simulink model "entryVehicle"  (R2024b)
settings: Solver=ode5  StartTime=startTime  StopTime=stopTime  FixedStep=stepTime  RelTol=1e-3
values from neighbouring files (symbols this model uses):
  acce_bias = [0; 0; 0]    [run_entryVehicle.m]
  acce_S = [0, 0, 0 ... (first row only)    [run_entryVehicle.m]
  alpha_0 = deg2rad(-23.82)    [run_entryVehicle.m]
  beta_0 = deg2rad(0.0)    [run_entryVehicle.m]
  chi_0 = deg2rad(90)    [run_entryVehicle.m]
  d_ref = 3.9    [run_entryVehicle.m]
  gamma_0 = deg2rad(-9.536)    [run_entryVehicle.m]
  H_s = 7050    [run_entryVehicle.m]
  I_xx = 5617.61    [run_entryVehicle.m]
  I_xz = 0    [run_entryVehicle.m]
  I_yy = 4454.62    [run_entryVehicle.m]
  I_zz = 4454.80    (= 4454.8)    [run_entryVehicle.m]
  lambda_0 = deg2rad(0)    [run_entryVehicle.m]
  m_0 = 4976    [run_entryVehicle.m]
  Mars_radius = 6371e3    (= 6371000)    [run_entryVehicle.m]
  p_0 = deg2rad(0)    [run_entryVehicle.m]
  Q0 = [Q1; Q2; Q3; Q4]    [get_Q0.m]    (also in run_entryVehicle.m = get_Q0(tau_0, lambda_0, chi_0, gamma_0, alpha_0, beta_0, sig)
  q_0 = deg2rad(0)    [run_entryVehicle.m]
  r0_eci = [x; y; z]    [getInitialECI.m]
  r_0 = deg2rad(0)    [run_entryVehicle.m]
  R_0 = 220e3 + Mars_radius    (= 6591000)    [run_entryVehicle.m]
  r_cm = [-0.137; 0; 1.8]    [run_entryVehicle.m]
  R_s = 287    [run_entryVehicle.m]
  rateGyro_bias = [0; 0; 0]    [run_entryVehicle.m]
  rateGyro_S = [0, 0, 0 ... (first row only)    [run_entryVehicle.m]
  rho_0 = 1.225    [run_entryVehicle.m]
  S_ref = 12    [run_entryVehicle.m]
  sigma_0 = deg2rad(100.)    [run_entryVehicle.m]
  specific_heat = 1.29    [run_entryVehicle.m]
  stepTime = 0.01    [run_entryVehicle.m]
  tau_0 = deg2rad(0)    [run_entryVehicle.m]
  v0_eci = T_ECI_NED * v_ned    [getInitialECI.m]
  V_0 = 11e3    (= 11000)    [run_entryVehicle.m]
undefined symbols (not defined in the file or in its folder): A_attitude, alpha_T_CD, alpha_T_CL, alpha_T_Cm, alpha_T_Cm_q, B_attitude, CD_T, CL_T, Cm_qT, Cm_T, K_lat, K_long, lateral_ref, longitudinal_ref, Mach_numbers_CD, Mach_numbers_CL, Mach_numbers_Cm, Mach_numbers_Cm_q, Mars_mu, my_max
libraries: simulink_extras x33, aerolibnav x2, simulink x1, SignalEditorBlockLib x1
(part 1 of 2)
settings Model: Creator=tester  LastModifiedBy=rafae

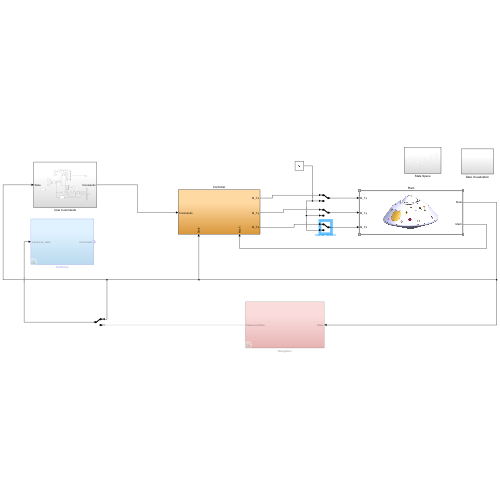
[thumbnail: Simulink's stored preview of the top-level diagram]
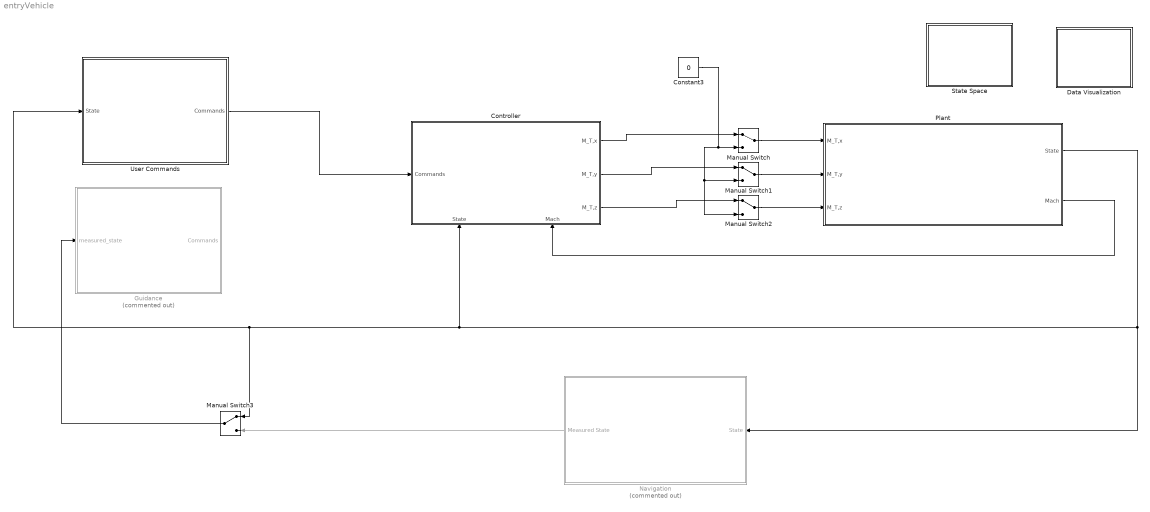
== system entryVehicle ==
  Constant3 : Constant  Value=0
  Controller : Subsystem
      settings: PortSchema="{\"entries\":[{\"content\":{\"sides\":[{\"content\":{\"connectorIds\":[\"In1\"]},\"type\":\"ConnectorPlacement.EquallySpacedRectSide\",\"uuid\":\"6730c763-0db7-4539-af59-842a5691e68e\"},{\"content\":{\"connectorIds\":[\"Out1\",\"Out2\",\"Out3\"],\"side\":\"RIGHT\"},\"type\":\"ConnectorPlacement.EquallySpacedRectSide\",\"uuid\":\"60c274f5-9a0e-4442-9031-a8a2f12bc615\"},{\"content\":{\"side\":\"TOP\"},\"type\":\"ConnectorPlacement.EquallySpacedRectSide\",\"uuid\":\"e1e9f683-9b0b-4096-8ce5-6b557ad43515\"},{\"content\":{\"connectorIds\":[\"In2\",\"In3\"],\"side\":\"BOTTOM\"},\"type\":\"ConnectorPlacement.EquallySpacedRectSide\",\"uuid\":\"b92da982-2d47-4e6b-9095-2c7c1889c431\"}]},\"type\":\"ConnectorPlacement.EquallySpacedConnector\",\"uuid\":\"278978b4-8d2f-4edc-bb2a-9785bc810a53\"}],\"packageUris\":[\"http://schema.mathworks.com/mf0/Connector/R2020b\"],\"version\":\"1.0\"}"
  Data Visualization : Subsystem
  Guidance : Subsystem  Commented=on
  Manual Switch{,1..3} (4 alike) : ManualSwitch
  Navigation : Subsystem  Commented=on
  Plant : Subsystem
      mask Display: image('MSLEntryVehicle.jpg', [0,0,0,0,100,90]);
  State Space : Subsystem
  User Commands : Subsystem
  wires:
  Controller/1(M_T,x) -> Manual Switch/1
  Manual Switch/1 -> Plant/1(M_T,x)
  Manual Switch2/1 -> Plant/3(M_T,z)
  Manual Switch1/1 -> Plant/2(M_T,y)
  Controller/2(M_T,y) -> Manual Switch1/1
  Controller/3(M_T,z) -> Manual Switch2/1
  Constant3/1 -> Manual Switch1/2, Manual Switch2/2, Manual Switch/2
  Plant/1(State) -> Controller/2(State), Manual Switch3/1, User Commands/1(State), Navigation/1(State)
  Plant/2(Mach) -> Controller/3(Mach)
  Navigation/1(Measured State) -> Manual Switch3/2
  Manual Switch3/1 -> Guidance/1(measured_state)
  User Commands/1(Commands) -> Controller/1(Commands)

== system entryVehicle/Controller ==
  note: Lateral Controller
  note: Longitudinal Controller
  Commands : Inport
  State : Inport  Port=2
  Mach : Inport  Port=3
  Demux : Demux  Outputs=6
  Demux1 : Demux  Outputs=2
  Integrator Subsystem : Subsystem
  Integrator Subsystem1 : Subsystem
  Lateral Gain Scheduling : Subsystem
  Lateral Input : Subsystem
  Longitude Gain Scheduling : Subsystem
  Longitudinal Input : Subsystem
  Matrix Multiply : Product  Multiplication=Matrix(*)
  Matrix Multiply1 : Product  Multiplication=Matrix(*)
  Scope : Scope
  Scope1 : Scope
  Subsystem : Subsystem
  Subtract : Sum  Inputs=+-
  Sum : Sum  Inputs=|++
  Sum1 : Sum  Inputs=|++
  M_T,x : Outport
  M_T,y : Outport  Port=2
  M_T,z : Outport  Port=3
  wires:
  State/1 -> Subsystem/1(State)
  Demux/1 -> Integrator Subsystem1/1(Delta_alpha), Longitudinal Input/2(Delta_alpha)
  Demux/5 -> Longitudinal Input/1(Delta_q)
  Demux/2 -> Lateral Input/3(Delta_beta)
  Demux/3 -> Lateral Input/4(Delta_sigma), Integrator Subsystem/1(Delta_sigma)
  Demux/4 -> Lateral Input/1(Delta_p)
  Demux/6 -> Lateral Input/2(Delta_r)
  Commands/1 -> Subtract/2
  Subtract/1 -> Demux/1
  Subsystem/1(Feedback) -> Subtract/1
  Mach/1 -> Longitude Gain Scheduling/1(Mach), Integrator Subsystem1/2(Mach), Integrator Subsystem/2(Mach), Lateral Gain Scheduling/1(Mach)
  Longitudinal Input/1(Longitudinal_error) -> Matrix Multiply1/1
  Longitude Gain Scheduling/1(Longitude Gain) -> Matrix Multiply1/2, Scope/1
  Lateral Gain Scheduling/1(Lateral Gain) -> Matrix Multiply/1
  Matrix Multiply/1 -> Demux1/1
  Demux1/1 -> Sum/1
  Sum/1 -> Scope1/1, M_T,x/1
  Matrix Multiply1/1 -> Sum1/1
  Sum1/1 -> M_T,y/1
  Integrator Subsystem1/1(integrator_term) -> Sum1/2
  Integrator Subsystem/1(integrator_term) -> Sum/2
  Demux1/2 -> M_T,z/1
  Lateral Input/1(Lateral_error) -> Matrix Multiply/2

== system entryVehicle/Data Visualization ==

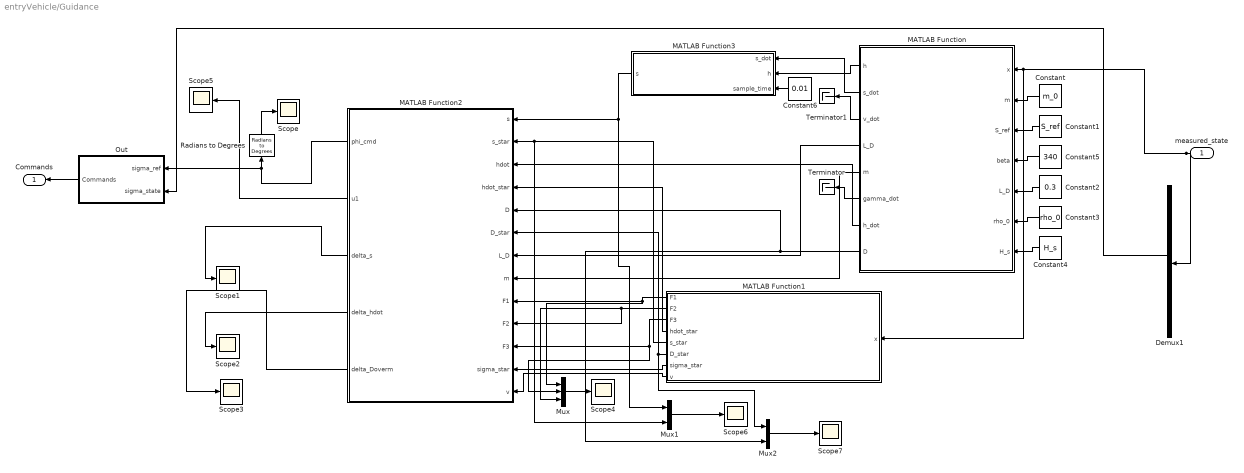
== system entryVehicle/Guidance ==
  measured_state : Inport
  Constant : Constant  Value=m_0
  Constant1 : Constant  Value=S_ref
  Constant2 : Constant  Value=0.3
  Constant3 : Constant  Value=rho_0
  Constant4 : Constant  Value=H_s
  Constant5 : Constant  Value=340
  Constant6 : Constant  Value=0.01
  Demux1 : Demux  Outputs=12
  MATLAB Function : MATLAB Function  TreatAsAtomicUnit=on
  MATLAB Function1 : MATLAB Function  TreatAsAtomicUnit=on
  MATLAB Function2 : MATLAB Function  TreatAsAtomicUnit=on
  MATLAB Function3 : MATLAB Function  TreatAsAtomicUnit=on  SystemSampleTime=0.01
  Mux : Mux  Inputs=3
  Mux1 : Mux  Inputs=2
  Mux2 : Mux  Inputs=2
  Out : Subsystem
  Radians to Degrees : simulink_extras/Transformations/Radians to Degrees
  Scope{,1..7} (8 alike) : Scope
  Terminator : Terminator
  Terminator1 : Terminator
  Commands : Outport
  wires:
  Constant/1 -> MATLAB Function/2("m ")
  Constant1/1 -> MATLAB Function/3(S_ref)
  Constant2/1 -> MATLAB Function/5("L_D ")
  Constant3/1 -> MATLAB Function/6(rho_0)
  Constant4/1 -> MATLAB Function/7(H_s)
  Constant5/1 -> MATLAB Function/4(beta)
  measured_state/1 -> MATLAB Function1/1(x), MATLAB Function/1(x), Demux1/1
  MATLAB Function/7(h_dot) -> MATLAB Function2/3(hdot)
  MATLAB Function/5(m) -> MATLAB Function2/8(m)
  MATLAB Function/4(L_D) -> MATLAB Function2/7(L_D)
  MATLAB Function/8(D) -> Mux2/2, MATLAB Function2/5(D)
  MATLAB Function/6(gamma_dot) -> Terminator/1
  MATLAB Function/3(v_dot) -> Terminator1/1
  MATLAB Function1/1(F1) -> Mux/1, MATLAB Function2/9(F1)
  MATLAB Function1/2(F2) -> Mux/3, MATLAB Function2/10(F2)
  MATLAB Function1/3(F3) -> Mux/2, MATLAB Function2/11(F3)
  MATLAB Function1/4(hdot_star) -> MATLAB Function2/4(hdot_star)
  MATLAB Function1/5(s_star) -> Mux1/2, MATLAB Function2/2(s_star)
  MATLAB Function1/6(D_star) -> Mux2/1, MATLAB Function2/6(D_star)
  MATLAB Function1/7(sigma_star) -> MATLAB Function2/12(sigma_star)
  Radians to Degrees/1 -> Scope/1
  MATLAB Function/2(s_dot) -> MATLAB Function3/1(s_dot)
  MATLAB Function/1(h) -> MATLAB Function3/2(h)
  MATLAB Function3/1(s) -> MATLAB Function2/1(s), Mux1/1
  MATLAB Function1/8(v) -> MATLAB Function2/13(v)
  MATLAB Function2/3(delta_s) -> Scope1/1
  Mux/1 -> Scope4/1
  MATLAB Function2/2(u1) -> Scope5/1
  Mux1/1 -> Scope6/1
  MATLAB Function2/4(delta_hdot) -> Scope2/1
  MATLAB Function2/5(delta_Doverm) -> Scope3/1
  Constant6/1 -> MATLAB Function3/3(sample_time)
  Mux2/1 -> Scope7/1
  MATLAB Function2/1(phi_cmd) -> Radians to Degrees/1, Out/1(sigma_ref)
  Out/1(Commands) -> Commands/1
  Demux1/6 -> Out/2(sigma_state)

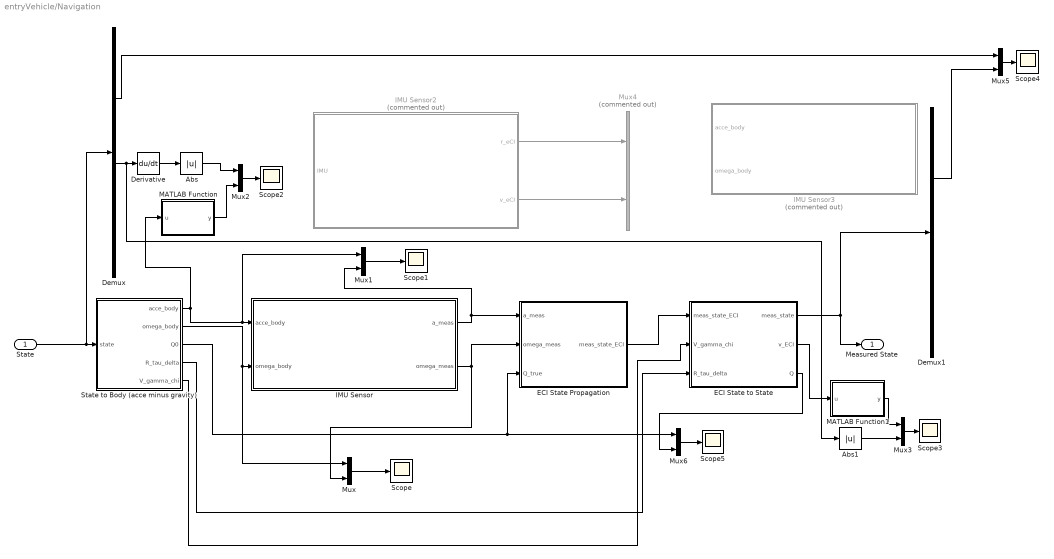
== system entryVehicle/Navigation ==
  State : Inport
  Abs : Abs  SaturateOnIntegerOverflow=off
  Abs1 : Abs  SaturateOnIntegerOverflow=off
  Demux : Demux  Outputs=12
  Demux1 : Demux  Outputs=12
  Derivative : Derivative
  ECI State Propagation : Subsystem
  ECI State to State : Subsystem
  IMU Sensor : Subsystem
  IMU Sensor2 : Subsystem  Commented=on
  IMU Sensor3 : Subsystem  Commented=on
  MATLAB Function : MATLAB Function  TreatAsAtomicUnit=on
  MATLAB Function1 : MATLAB Function  TreatAsAtomicUnit=on
  Mux{,1..3,5..6} (6 alike) : Mux  Inputs=2
  Mux4 : Mux  Commented=on  Inputs=2
  Scope{,1..5} (6 alike) : Scope
  State to Body (acce minus gravity) : Subsystem
  Measured State : Outport
  wires:
  IMU Sensor2/2(v_eCI) -> Mux4/2
  IMU Sensor2/1(r_eCI) -> Mux4/1
  State/1 -> Demux/1, State to Body (acce minus gravity)/1(state)
  ECI State to State/1(meas_state) -> Measured State/1, Demux1/1
  State to Body (acce minus gravity)/1(acce_body) -> Mux1/1, IMU Sensor/1(acce_body), MATLAB Function/1(u)
  State to Body (acce minus gravity)/2(omega_body) -> Mux/1, IMU Sensor/2(omega_body)
  IMU Sensor/1(a_meas) -> Mux1/2, ECI State Propagation/1(a_meas)
  IMU Sensor/2(omega_meas) -> Mux/2, ECI State Propagation/2(omega_meas)
  ECI State Propagation/1(meas_state_ECI) -> ECI State to State/1(meas_state_ECI)
  Mux/1 -> Scope/1
  Mux1/1 -> Scope1/1
  Abs/1 -> Mux2/1
  MATLAB Function/1(y) -> Mux2/2
  Mux2/1 -> Scope2/1
  Derivative/1 -> Abs/1
  ECI State to State/2(v_ECI) -> MATLAB Function1/1(u)
  MATLAB Function1/1(y) -> Mux3/1
  Mux3/1 -> Scope3/1
  Abs1/1 -> Mux3/2
  Demux/7 -> Abs1/1, Derivative/1
  Demux1/4 -> Mux5/2
  Mux5/1 -> Scope4/1
  Demux/4 -> Mux5/1
  State to Body (acce minus gravity)/3(Q0) -> ECI State Propagation/3(Q_true), Mux6/1
  ECI State to State/3(Q) -> Mux6/2
  Mux6/1 -> Scope5/1
  State to Body (acce minus gravity)/4(R_tau_delta) -> ECI State to State/3(R_tau_delta)
  State to Body (acce minus gravity)/5(V_gamma_chi) -> ECI State to State/2(V_gamma_chi)

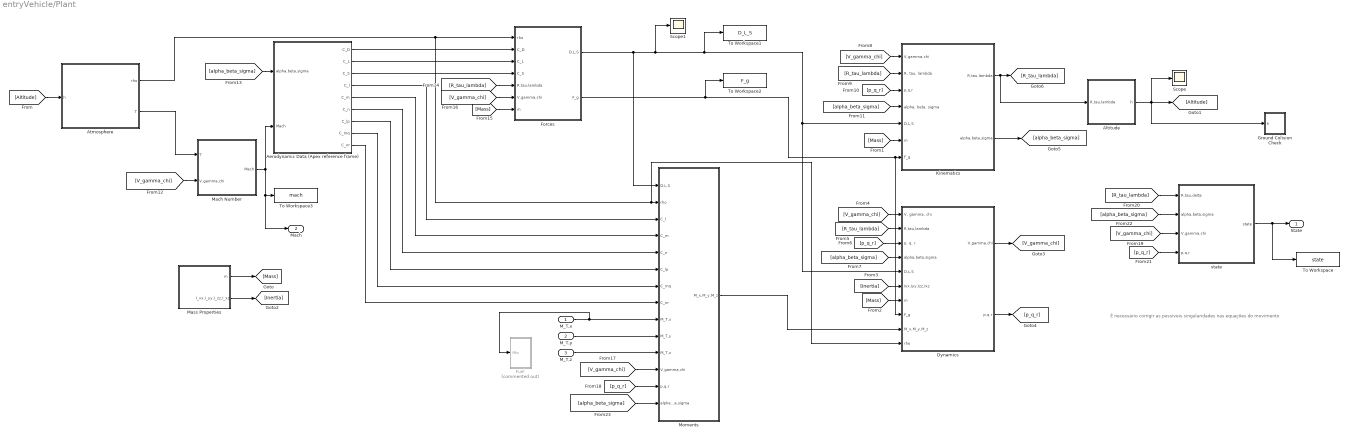
== system entryVehicle/Plant ==
  note: É necessário corrigir as possíveis singularidades nas equações do movimento
  M_T,x : Inport
  M_T,y : Inport  Port=2
  M_T,z : Inport  Port=3
  Aerodynamic Data (Apex reference frame) : Subsystem
  Altitude : Subsystem
  Atmosphere : Subsystem
  Dynamics : Subsystem
  Forces : Subsystem
  Fuel : Subsystem  Commented=on
  Ground Colision Check : Subsystem
  Kinematics : Subsystem
  Mach Number : Subsystem
  Mass Properties : Subsystem
  Moments : Subsystem
  Scope : Scope
  Scope1 : Scope
  To Workspace : ToWorkspace  VariableName=state  SaveFormat=Structure With Time  SampleTime=-1
  To Workspace1 : ToWorkspace  VariableName=D_L_S  SaveFormat=Structure With Time  SampleTime=-1
  To Workspace2 : ToWorkspace  VariableName=F_g  SaveFormat=Structure With Time  SampleTime=-1
  To Workspace3 : ToWorkspace  VariableName=mach  SaveFormat=Structure With Time  SampleTime=-1
  state : Subsystem
  State : Outport
  Mach : Outport  Port=2
  wires:
  M_T,x/1 -> Fuel/1(Mtx), Moments/9(M_T,x)
  M_T,y/1 -> Moments/10(M_T,y)
  M_T,z/1 -> Moments/11(M_T,z)
  Aerodynamic Data (Apex reference frame)/6(C_n) -> Moments/5(C_n)
  Aerodynamic Data (Apex reference frame)/5(C_m) -> Moments/4(C_m)
  Aerodynamic Data (Apex reference frame)/4(C_l) -> Moments/3(C_l)
  Altitude/1(h) -> [Altitude], Scope/1, Ground Colision Check/1(h)
  [Altitude] -> Atmosphere/1(h)
  Mass Properties/1(m) -> [Mass]
  [Mass] -> Kinematics/6(m)
  Mass Properties/2(I_xx,I_yy,I_zz,I_xz) -> [Inertia]
  Forces/2(F_g) -> To Workspace2/1, Dynamics/8(F_g), Kinematics/7(F_g)
  [Mass] -> Dynamics/7(m)
  [Inertia] -> Dynamics/6(Ixx,Iyy,Izz,Ixz)
  Forces/1(D,L,S) -> Scope1/1, To Workspace1/1, Dynamics/5(D,L,S), Kinematics/5(D,L,S), Moments/1(D,L,S)
  Moments/1(M_x,M_y,M_z) -> Dynamics/9(M_x,M_y,M_z)
  Dynamics/2(p,q,r) -> [p_q_r]
  Dynamics/1(V,gamma,chi) -> [V_gamma_chi]
  Kinematics/2(alpha,beta,sigma) -> [alpha_beta_sigma]
  [V_gamma_chi] -> Dynamics/1("V, gamma, chi")
  [R_tau_lambda] -> Dynamics/2(R,tau,lambda)
  Kinematics/1(R,tau,lambda) -> [R_tau_lambda], Altitude/1(R,tau,lambda)
  [p_q_r] -> Dynamics/3("p, q, r")
  [alpha_beta_sigma] -> Dynamics/4(alpha,beta,sigma)
  [V_gamma_chi] -> Kinematics/1(V,gamma,chi)
  [R_tau_lambda] -> Kinematics/2("R, tau, lambda")
  [p_q_r] -> Kinematics/3(p,q,r)
  [alpha_beta_sigma] -> Kinematics/4("alpha, beta, sigma")
  Mach Number/1(Mach) -> To Workspace3/1, Mach/1, Aerodynamic Data (Apex reference frame)/2(Mach)
  [V_gamma_chi] -> Mach Number/2(V,gamma,chi)
  Atmosphere/1(rho) -> Dynamics/10(rho), Moments/2(rho), Forces/1(rho)
  [alpha_beta_sigma] -> Aerodynamic Data (Apex reference frame)/1(alpha,beta,sigma)
  [R_tau_lambda] -> Forces/5(R,tau,lambda)
  [Mass] -> Forces/7(m)
  [V_gamma_chi] -> Forces/6(V,gamma,chi)
  [V_gamma_chi] -> Moments/12(V,gamma,chi)
  Atmosphere/2(T) -> Mach Number/1(T)
  Aerodynamic Data (Apex reference frame)/1(C_D) -> Forces/2(C_D)
  Aerodynamic Data (Apex reference frame)/2(C_L) -> Forces/3(C_L)
  Aerodynamic Data (Apex reference frame)/3(C_S) -> Forces/4(C_S)
  [p_q_r] -> Moments/13(p,q,r)
  Aerodynamic Data (Apex reference frame)/9(C_nr) -> Moments/8(C_nr)
  Aerodynamic Data (Apex reference frame)/8(C_mq) -> Moments/7(C_mq)
  Aerodynamic Data (Apex reference frame)/7(C_lp) -> Moments/6(C_lp)
  [V_gamma_chi] -> state/3(V,gamma,chi)
  [R_tau_lambda] -> state/1(R,tau,delta)
  [p_q_r] -> state/4(p,q,r)
  [alpha_beta_sigma] -> state/2(alpha,beta,sigma)
  state/1(state) -> To Workspace/1, State/1
  [alpha_beta_sigma] -> Moments/14(alpha,beta,sigma)

== system entryVehicle/State Space ==
  Demux : Demux  Commented=on  Outputs=6
  Gain : Gain  Commented=on  Gain=my_max
  Lateral_Controller : Subsystem  Commented=on
  Longitudinal_Controller : Subsystem  Commented=on
  MATLAB Function : MATLAB Function  Commented=on  TreatAsAtomicUnit=on
  Mux1 : Mux  Commented=on
  Mux2 : Mux  Commented=on  Inputs=2
  Radians to Degrees{1..5} (5 alike) : simulink_extras/Transformations/Radians to Degrees  Commented=on
  References : Subsystem  Commented=on
  Scope{1..7} (7 alike) : Scope  Commented=on
  State-Space : StateSpace  Commented=on  A=A_attitude  B=B_attitude  C=eye(6)  D=zeros(6,3)  InitialCondition=[0; 0; 0; -0.101; 0; 0]
  alpha_deg : simulink_extras/Transformations/Radians to Degrees  Commented=on
  wires:
  Radians to Degrees1/1 -> Scope3/1
  MATLAB Function/1(u) -> Scope7/1, State-Space/1
  Demux/4 -> alpha_deg/1, Mux2/2  "alpha"
  Radians to Degrees2/1 -> Scope4/1
  Lateral_Controller/1(Mx,Mtz) -> MATLAB Function/2(Mtx_Mtz)
  Demux/1 -> Mux1/1, Radians to Degrees5/1  "p"
  Longitudinal_Controller/1(My) -> Gain/1
  Demux/3 -> Mux1/2, Radians to Degrees3/1  "r"
  Demux/2 -> Mux2/1, Radians to Degrees4/1  "q"
  Demux/5 -> Mux1/3, Radians to Degrees1/1  "beta"
  Radians to Degrees3/1 -> Scope6/1
  Radians to Degrees5/1 -> Scope1/1
  Radians to Degrees4/1 -> Scope5/1
  Demux/6 -> Mux1/4, Radians to Degrees2/1  "sigma"
  State-Space/1 -> Demux/1
  alpha_deg/1 -> Scope2/1
  References/1(out_longitudinal ref) -> Longitudinal_Controller/2(longitudinal_ref)
  Mux1/1 -> Lateral_Controller/1(lateral_state)
  References/2(out_lateral_ref) -> Lateral_Controller/2(lateral_ref)
  Gain/1 -> MATLAB Function/1(My)
  Mux2/1 -> Longitudinal_Controller/1(longitudinal)

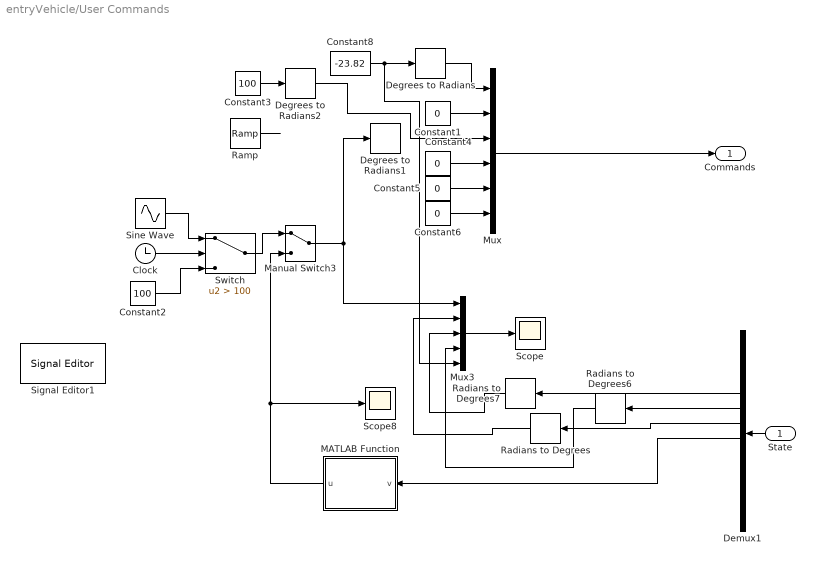
== system entryVehicle/User Commands ==
  State : Inport
  Clock : Clock
  Constant{1,4..6} (4 alike) : Constant  Value=0
  Constant2 : Constant  Value=100
  Constant3 : Constant  Value=100
  Constant8 : Constant  Value=-23.82
  Degrees to Radians : simulink_extras/Transformations/Degrees to Radians
  Degrees to Radians1 : simulink_extras/Transformations/Degrees to Radians
  Degrees to Radians2 : simulink_extras/Transformations/Degrees to Radians
  Demux1 : Demux  Outputs=12
  MATLAB Function : MATLAB Function  TreatAsAtomicUnit=on
  Manual Switch3 : ManualSwitch
  Mux : Mux  Inputs=6
  Mux3 : Mux  Inputs=5
  Radians to Degrees : simulink_extras/Transformations/Radians to Degrees
  Radians to Degrees6 : simulink_extras/Transformations/Radians to Degrees
  Radians to Degrees7 : simulink_extras/Transformations/Radians to Degrees
  Ramp : simulink/Sources/Ramp  slope=1  start=100  InitialOutput=70
  Scope : Scope
  Scope8 : Scope
  Signal Editor1 : SignalEditorBlockLib/Signal Editor  FileName=sigma_ref_dataset.mat  ActiveScenario=signalDataset  ActiveSignal=sigma_ref  IsBus=off  OutputBusObjectStr=Bus: BusObject  SampleTime=0  Interpolate=off  ZeroCross=off  OutputAfterFinalValue=Setting to zero  Unit=inherit  PreserveSignalName=on  ApplySigPropsToAllScenarios=on  ApplySigPropsToAllSignals=off
  Sine Wave : Sin  Amplitude=20  Bias=100  Frequency=0.05  Phase=1.2  SampleTime=0
  Switch : Switch  Criteria=u2 > Threshold  Threshold=100  SaturateOnIntegerOverflow=off  InputSameDT=off
  Commands : Outport
  wires:
  MATLAB Function/1(u) -> Manual Switch3/2, Scope8/1
  Radians to Degrees/1 -> Mux3/2
  Constant5/1 -> Mux/5
  Ramp/1 -> ?
  State/1 -> Demux1/1
  Constant4/1 -> Mux/4
  Sine Wave/1 -> Switch/1
  Constant6/1 -> Mux/6
  Demux1/5 -> Radians to Degrees6/1
  Radians to Degrees7/1 -> Mux3/3
  Constant2/1 -> Switch/3
  Degrees to Radians/1 -> Mux/1
  Mux/1 -> Commands/1
  Constant8/1 -> Mux3/5, Degrees to Radians/1
  Switch/1 -> Manual Switch3/1
  Manual Switch3/1 -> Mux3/1, Degrees to Radians1/1
  Mux3/1 -> Scope/1
  Demux1/4 -> Radians to Degrees7/1
  Demux1/6 -> Radians to Degrees/1
  Clock/1 -> Switch/2
  Constant1/1 -> Mux/2
  Radians to Degrees6/1 -> Mux3/4
  Demux1/7 -> MATLAB Function/1(v)
  Constant3/1 -> Degrees to Radians2/1
  Degrees to Radians2/1 -> Mux/3

== system entryVehicle/Controller/Integrator Subsystem ==
  Delta_sigma : Inport
  Mach : Inport  Port=2
  Gain : Gain
  Integrator : Integrator
  MATLAB Function : MATLAB Function  TreatAsAtomicUnit=on
  Product : Product
  Scope : Scope
  integrator_term : Outport
  wires:
  Delta_sigma/1 -> Integrator/1
  Mach/1 -> MATLAB Function/1(Mach)
  Integrator/1 -> Product/1
  MATLAB Function/1(K_integrator_sigma) -> Scope/1, Gain/1
  Product/1 -> integrator_term/1
  Gain/1 -> Product/2

== system entryVehicle/Controller/Integrator Subsystem1 ==
  Delta_alpha : Inport
  Mach : Inport  Port=2
  Gain : Gain  Gain=-1
  Integrator : Integrator
  MATLAB Function : MATLAB Function  TreatAsAtomicUnit=on
  Product : Product
  Scope : Scope
  integrator_term : Outport
  wires:
  Delta_alpha/1 -> Integrator/1
  Mach/1 -> MATLAB Function/1(Mach)
  Integrator/1 -> Product/1
  MATLAB Function/1(K_integrator_alpha) -> Gain/1, Scope/1
  Product/1 -> integrator_term/1
  Gain/1 -> Product/2

== system entryVehicle/Controller/Lateral Gain Scheduling ==
  Mach : Inport
  Gain : Gain  Gain=-1
  MATLAB Function : MATLAB Function  TreatAsAtomicUnit=on
  Lateral Gain : Outport
  wires:
  Mach/1 -> MATLAB Function/1(Mach)
  Gain/1 -> Lateral Gain/1
  MATLAB Function/1(K_lat) -> Gain/1

== system entryVehicle/Controller/Lateral Input ==
  Delta_p : Inport
  Delta_r : Inport  Port=2
  Delta_beta : Inport  Port=3
  Delta_sigma : Inport  Port=4
  Mux : Mux
  Transpose : Math  Operator=transpose
  Lateral_error : Outport
  wires:
  Mux/1 -> Transpose/1
  Delta_r/1 -> Mux/2
  Delta_beta/1 -> Mux/3
  Transpose/1 -> Lateral_error/1
  Delta_p/1 -> Mux/1
  Delta_sigma/1 -> Mux/4

== system entryVehicle/Controller/Longitude Gain Scheduling ==
  Mach : Inport
  Gain : Gain  Gain=-1
  MATLAB Function : MATLAB Function  TreatAsAtomicUnit=on
  Longitude Gain : Outport
  wires:
  Mach/1 -> MATLAB Function/1(Mach)
  MATLAB Function/1(K_long) -> Gain/1
  Gain/1 -> Longitude Gain/1

== system entryVehicle/Controller/Longitudinal Input ==
  Delta_q : Inport
  Delta_alpha : Inport  Port=2
  Mux : Mux  Inputs=2
  Transpose1 : Math  Operator=transpose
  Longitudinal_error : Outport
  wires:
  Delta_q/1 -> Mux/1
  Delta_alpha/1 -> Mux/2
  Mux/1 -> Transpose1/1
  Transpose1/1 -> Longitudinal_error/1

== system entryVehicle/Controller/Subsystem ==
  State : Inport
  Demux : Demux  Outputs=12
  Mux : Mux  Inputs=6
  Feedback : Outport
  wires:
  State/1 -> Demux/1
  Mux/1 -> Feedback/1
  Demux/4 -> Mux/1  "alpha"
  Demux/5 -> Mux/2  "beta"
  Demux/6 -> Mux/3  "sigma"
  Demux/10 -> Mux/4  "p"
  Demux/12 -> Mux/6  "r"
  Demux/11 -> Mux/5  "q"

== system entryVehicle/Guidance/Out ==
  sigma_ref : Inport
  sigma_state : Inport  Port=2
  Constant{7,9..11} (4 alike) : Constant  Value=0
  Constant8 : Constant  Value=-23.82
  Degrees to Radians : simulink_extras/Transformations/Degrees to Radians
  Mux : Mux  Inputs=2
  Mux3 : Mux  Inputs=6
  Scope : Scope
  Commands : Outport
  wires:
  Constant7/1 -> Mux3/2
  Constant11/1 -> Mux3/6
  Mux3/1 -> Commands/1
  Constant8/1 -> Degrees to Radians/1
  Constant10/1 -> Mux3/5
  Degrees to Radians/1 -> Mux3/1
  Constant9/1 -> Mux3/4
  sigma_ref/1 -> Mux/1, Mux3/3
  sigma_state/1 -> Mux/2
  Mux/1 -> Scope/1

== system entryVehicle/Navigation/ECI State Propagation ==
  note: Inertial Position Propagation
  note: Inertial Velocity Propagation
  note: Intertial Attitude Propagation
  a_meas : Inport
  omega_meas : Inport  Port=2
  Q_true : Inport  Port=3
  Constant : Constant  Value=Mars_mu
  Integrator3 : Integrator  InitialCondition=Q0
  Integrator4 : Integrator  InitialCondition=v0_eci
  Integrator5 : Integrator  InitialCondition=r0_eci
  MATLAB Function : MATLAB Function  TreatAsAtomicUnit=on
  MATLAB Function1 : MATLAB Function  TreatAsAtomicUnit=on
  MATLAB Function2 : MATLAB Function  TreatAsAtomicUnit=on
  MATLAB Function3 : MATLAB Function  TreatAsAtomicUnit=on
  Mux : Mux
  Product1 : Product  Multiplication=Matrix(*)
  Scope : Scope
  Sum1 : Sum  Inputs=|++
  meas_state_ECI : Outport
  wires:
  omega_meas/1 -> MATLAB Function2/2(omega), Mux/4  "omega_meas"
  Integrator3/1 -> MATLAB Function/1(Q_in)
  MATLAB Function1/1(TIC) -> Product1/1
  a_meas/1 -> Product1/2
  Product1/1 -> Sum1/1
  Sum1/1 -> Integrator4/1
  Integrator4/1 -> Mux/2, Integrator5/1  "v_meas_ECI"
  Integrator5/1 -> MATLAB Function3/1(r_ECI), Mux/1  "r_meas_ECI"
  Mux/1 -> meas_state_ECI/1
  MATLAB Function3/1(g_vec_ECI) -> Scope/1, Sum1/2
  Constant/1 -> MATLAB Function3/2(mu)
  MATLAB Function2/1(Q_dot) -> Integrator3/1
  MATLAB Function/1(Q_out) -> Mux/3, MATLAB Function2/1(Q)  "Q_meas_ECI"
  Q_true/1 -> MATLAB Function1/1(Q)

== system entryVehicle/Navigation/ECI State to State ==
  meas_state_ECI : Inport
  V_gamma_chi : Inport  Port=2
  R_tau_delta : Inport  Port=3
  Demux : Demux  Outputs=13
  Demux1 : Demux  Outputs=3
  MATLAB Function : MATLAB Function  TreatAsAtomicUnit=on
  MATLAB Function1 : MATLAB Function  TreatAsAtomicUnit=on
  MATLAB Function2 : MATLAB Function  TreatAsAtomicUnit=on
  MATLAB Function3 : MATLAB Function  TreatAsAtomicUnit=on
  Mux : Mux  Inputs=3
  Mux1 : Mux  Inputs=3
  Mux2 : Mux
  Mux3 : Mux  Inputs=3
  Mux4 : Mux
  Mux5 : Mux  Inputs=2
  Scope : Scope
  meas_state : Outport
  v_ECI : Outport  Port=2
  Q : Outport  Port=3
  wires:
  meas_state_ECI/1 -> Demux/1
  Demux/2 -> Mux/2  "r_y"
  Demux/6 -> Mux1/3  "v_z"
  Demux/5 -> Mux1/2  "v_y"
  Demux/3 -> Mux/3  "r_z"
  Demux/1 -> Mux/1  "r_x"
  Demux/4 -> Mux1/1  "v_x"
  Demux/7 -> Mux2/1  "q1"
  Demux/8 -> Mux2/2  "q2"
  Demux/9 -> Mux2/3  "q3"
  Demux/10 -> Mux2/4  "q4"
  Mux/1 -> MATLAB Function/1(r_ECI)  "r_ECI"
  Mux1/1 -> v_ECI/1, MATLAB Function2/1(u), MATLAB Function1/1(v_ECI)  "v_ECI"
  Mux2/1 -> Q/1, MATLAB Function3/1(Q)  "Q"
  MATLAB Function1/1(V_gamma_chi) -> Demux1/1, Mux4/3
  MATLAB Function/1(R_tau_delta) -> MATLAB Function1/2(R_tau_delta), Mux4/1
  Demux/13 -> Mux3/3  "r"
  Demux/11 -> Mux3/1  "p"
  Demux/12 -> Mux3/2  "q"
  Mux4/1 -> meas_state/1
  MATLAB Function3/1(alpha_beta_sigma) -> Mux4/2
  Mux3/1 -> Mux4/4  "p_q_r"
  MATLAB Function2/1(y) -> Mux5/1
  Demux1/1 -> Mux5/2
  Mux5/1 -> Scope/1
  V_gamma_chi/1 -> MATLAB Function3/2(V_gamma_chi)
  R_tau_delta/1 -> MATLAB Function3/3(R_tau_delta)

== system entryVehicle/Navigation/IMU Sensor ==
  note: Rate Gyroscopes
  note: Accelerometers
  acce_body : Inport
  omega_body : Inport  Port=2
  Constant : Constant  Value=acce_bias
  Constant1 : Constant  Value=acce_S
  Constant2 : Constant  Value=rateGyro_bias
  Constant3 : Constant  Value=rateGyro_S
  MATLAB Function : MATLAB Function  TreatAsAtomicUnit=on
  MATLAB Function1 : MATLAB Function  TreatAsAtomicUnit=on
  a_meas : Outport
  omega_meas : Outport  Port=2
  wires:
  Constant/1 -> MATLAB Function/2(b_a)
  MATLAB Function/1(a_measured) -> a_meas/1
  acce_body/1 -> MATLAB Function/1(a_body)
  Constant1/1 -> MATLAB Function/3(S_a)
  omega_body/1 -> MATLAB Function1/1(omega_true)
  MATLAB Function1/1(omega_measured) -> omega_meas/1
  Constant3/1 -> MATLAB Function1/3(S_omega)
  Constant2/1 -> MATLAB Function1/2(b_gyro)

== system entryVehicle/Navigation/IMU Sensor2 ==
  IMU : Inport
  Constant : Constant  Value=[0;0;0]
  Constant1 : Constant  Value=[0, 0, 9.81]
  Demux : Demux
  Integrator : Integrator  InitialCondition=Q0
  Integrator1 : Integrator  InitialCondition=v0_eci
  Integrator2 : Integrator  InitialCondition=r0_eci
  MATLAB Function : MATLAB Function  TreatAsAtomicUnit=on
  MATLAB Function6 : MATLAB Function  TreatAsAtomicUnit=on
  MATLAB Function7 : MATLAB Function  TreatAsAtomicUnit=on
  Manual Switch : ManualSwitch
  Product : Product  Multiplication=Matrix(*)
  Radians to Degrees1 : simulink_extras/Transformations/Radians to Degrees
  Scope{,1..3,5} (5 alike) : Scope
  Sum : Sum  Inputs=|++
  Three-axis Inertial Measurement Unit : aerolibnav/Three-axis Inertial Measurement Unit  units=Metric (MKS)  imu=r_cm  i_Ts=0  dtype_a=on  w_a=190  z_a=0.707  a_sf_cc=[1 0 0; 0 1 0; 0 0 1]  a_bias=[0 0 0]  a_sat="[-inf  -inf  -inf  inf inf inf]"  dtype_g=on  w_g=190  z_g=0.707  g_sf_cc=[1 0 0; 0 1 0; 0 0 1]  g_bias=[0 0 0]  g_sens=[0 0 0]  g_sat="[-inf  -inf  -inf  inf inf inf]"  i_rand=on  i_seeds=[23093 23094 23095 23096 23097 23098]  i_pow=[1e-1 1e-1 1e-1 1e-7 1e-7 1e-7]
  Transpose : Math  Operator=transpose
  Transpose1 : Math  Operator=transpose
  r_eCI : Outport
  v_eCI : Outport  Port=2
  wires:
  IMU/1 -> Demux/1
  Demux/2 -> Three-axis Inertial Measurement Unit/1, Scope2/1
  Demux/3 -> Radians to Degrees1/1, Three-axis Inertial Measurement Unit/2
  Demux/4 -> Three-axis Inertial Measurement Unit/3
  Constant/1 -> Three-axis Inertial Measurement Unit/4
  Demux/1 -> Manual Switch/1, Scope3/1
  Manual Switch/1 -> Three-axis Inertial Measurement Unit/5
  Constant1/1 -> Manual Switch/2
  Radians to Degrees1/1 -> Scope5/1
  Three-axis Inertial Measurement Unit/2 -> MATLAB Function6/2(omega)
  MATLAB Function6/1(Q_dot) -> Integrator/1
  Integrator/1 -> MATLAB Function7/1(Q), MATLAB Function6/1(Q)
  Three-axis Inertial Measurement Unit/1 -> Transpose/1
  MATLAB Function7/1(TIC) -> Product/2
  Product/1 -> Sum/1
  Sum/1 -> Transpose1/1
  Integrator1/1 -> Scope/1, v_eCI/1, Integrator2/1
  Integrator2/1 -> MATLAB Function/1(r), Scope1/1, r_eCI/1
  Transpose/1 -> Product/1
  MATLAB Function/1(g_vec) -> Sum/2
  Transpose1/1 -> Integrator1/1

== system entryVehicle/Navigation/IMU Sensor3 ==
  acce_body : Inport
  omega_body : Inport  Port=2
  Constant : Constant  Value=[0;0;0]
  Constant1 : Constant  Value=[0, 0, 9.81]
  Demux : Demux
  Integrator : Integrator  InitialCondition=Q0
  Integrator1 : Integrator  InitialCondition=v0_eci
  Integrator2 : Integrator  InitialCondition=r0_eci
  MATLAB Function : MATLAB Function  TreatAsAtomicUnit=on
  MATLAB Function6 : MATLAB Function  TreatAsAtomicUnit=on
  MATLAB Function7 : MATLAB Function  TreatAsAtomicUnit=on
  Manual Switch : ManualSwitch
  Product : Product  Multiplication=Matrix(*)
  Radians to Degrees1 : simulink_extras/Transformations/Radians to Degrees
  Scope{,1..3,5} (5 alike) : Scope
  Sum : Sum  Inputs=|++
  Three-axis Inertial Measurement Unit : aerolibnav/Three-axis Inertial Measurement Unit  units=Metric (MKS)  imu=r_cm  i_Ts=0  dtype_a=on  w_a=190  z_a=0.707  a_sf_cc=[1 0 0; 0 1 0; 0 0 1]  a_bias=[0 0 0]  a_sat="[-inf  -inf  -inf  inf inf inf]"  dtype_g=on  w_g=190  z_g=0.707  g_sf_cc=[1 0 0; 0 1 0; 0 0 1]  g_bias=[0 0 0]  g_sens=[0 0 0]  g_sat="[-inf  -inf  -inf  inf inf inf]"  i_rand=on  i_seeds=[23093 23094 23095 23096 23097 23098]  i_pow=[1e-1 1e-1 1e-1 1e-7 1e-7 1e-7]
  Transpose : Math  Operator=transpose
  Transpose1 : Math  Operator=transpose
  wires:
  Transpose1/1 -> Integrator1/1
  MATLAB Function/1(g_vec) -> Sum/2
  Transpose/1 -> Product/1
  Integrator2/1 -> Scope1/1, MATLAB Function/1(r)
  Integrator1/1 -> Integrator2/1, Scope/1
  Sum/1 -> Transpose1/1
  Product/1 -> Sum/1
  MATLAB Function7/1(TIC) -> Product/2
  Three-axis Inertial Measurement Unit/1 -> Transpose/1
  Integrator/1 -> MATLAB Function6/1(Q), MATLAB Function7/1(Q)
  MATLAB Function6/1(Q_dot) -> Integrator/1
  Three-axis Inertial Measurement Unit/2 -> MATLAB Function6/2(omega)
  Radians to Degrees1/1 -> Scope5/1
  Constant1/1 -> Manual Switch/2
  Manual Switch/1 -> Three-axis Inertial Measurement Unit/5
  Demux/1 -> Scope3/1, Manual Switch/1
  Constant/1 -> Three-axis Inertial Measurement Unit/4
  Demux/4 -> Three-axis Inertial Measurement Unit/3
  Demux/3 -> Three-axis Inertial Measurement Unit/2, Radians to Degrees1/1
  Demux/2 -> Scope2/1, Three-axis Inertial Measurement Unit/1
  ? -> Demux/1

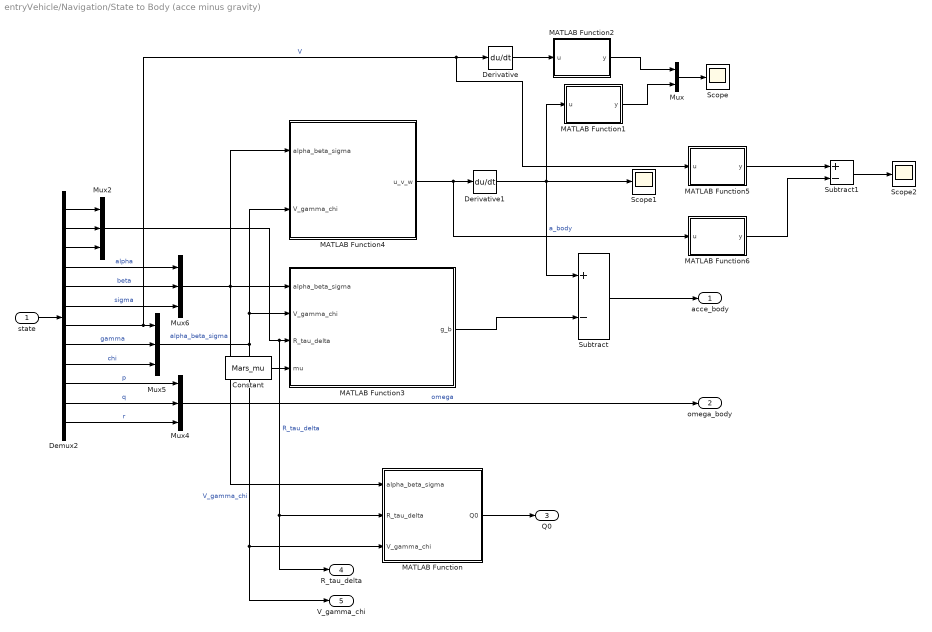
== system entryVehicle/Navigation/State to Body (acce minus gravity) ==
  state : Inport
  Constant : Constant  Value=Mars_mu
  Demux2 : Demux  Outputs=12
  Derivative : Derivative
  Derivative1 : Derivative
  MATLAB Function : MATLAB Function  TreatAsAtomicUnit=on
  MATLAB Function1 : MATLAB Function  TreatAsAtomicUnit=on
  MATLAB Function2 : MATLAB Function  TreatAsAtomicUnit=on
  MATLAB Function3 : MATLAB Function  TreatAsAtomicUnit=on
  MATLAB Function4 : MATLAB Function  TreatAsAtomicUnit=on
  MATLAB Function5 : MATLAB Function  TreatAsAtomicUnit=on
  MATLAB Function6 : MATLAB Function  TreatAsAtomicUnit=on
  Mux : Mux  Inputs=2
  Mux{2,4..6} (4 alike) : Mux  Inputs=3
  Scope : Scope
  Scope1 : Scope
  Scope2 : Scope
  Subtract : Sum  Inputs=+-
  Subtract1 : Sum  Inputs=+-
  acce_body : Outport
  omega_body : Outport  Port=2
  Q0 : Outport  Port=3
  R_tau_delta : Outport  Port=4
  V_gamma_chi : Outport  Port=5
  wires:
  state/1 -> Demux2/1
  Demux2/10 -> Mux4/1  "p"
  Demux2/11 -> Mux4/2  "q"
  Demux2/12 -> Mux4/3  "r"
  Demux2/7 -> Derivative/1, MATLAB Function5/1(u), Mux5/1  "V"
  Demux2/8 -> Mux5/2  "gamma"
  Demux2/9 -> Mux5/3  "chi"
  Demux2/4 -> Mux6/1  "alpha"
  Demux2/5 -> Mux6/2  "beta"
  Demux2/6 -> Mux6/3  "sigma"
  Mux4/1 -> omega_body/1  "omega"
  Mux5/1 -> MATLAB Function/3(V_gamma_chi), V_gamma_chi/1, MATLAB Function3/2(V_gamma_chi), MATLAB Function4/2(V_gamma_chi)  "V_gamma_chi"
  Mux6/1 -> MATLAB Function3/1(alpha_beta_sigma), MATLAB Function4/1(alpha_beta_sigma), MATLAB Function/1(alpha_beta_sigma)  "alpha_beta_sigma"
  Subtract/1 -> acce_body/1
  Demux2/2 -> Mux2/2
  Demux2/3 -> Mux2/3
  MATLAB Function4/1(u_v_w) -> Derivative1/1, MATLAB Function6/1(u)
  Derivative1/1 -> Subtract/1, Scope1/1, MATLAB Function1/1(u)  "a_body"
  MATLAB Function3/1(g_b) -> Subtract/2
  MATLAB Function1/1(y) -> Mux/2
  Derivative/1 -> MATLAB Function2/1(u)
  Mux/1 -> Scope/1
  MATLAB Function2/1(y) -> Mux/1
  MATLAB Function5/1(y) -> Subtract1/1
  MATLAB Function6/1(y) -> Subtract1/2
  Subtract1/1 -> Scope2/1
  Constant/1 -> MATLAB Function3/4(mu)
  Demux2/1 -> Mux2/1
  Mux2/1 -> MATLAB Function/2(R_tau_delta), R_tau_delta/1, MATLAB Function3/3(R_tau_delta)  "R_tau_delta"
  MATLAB Function/1(Q0) -> Q0/1

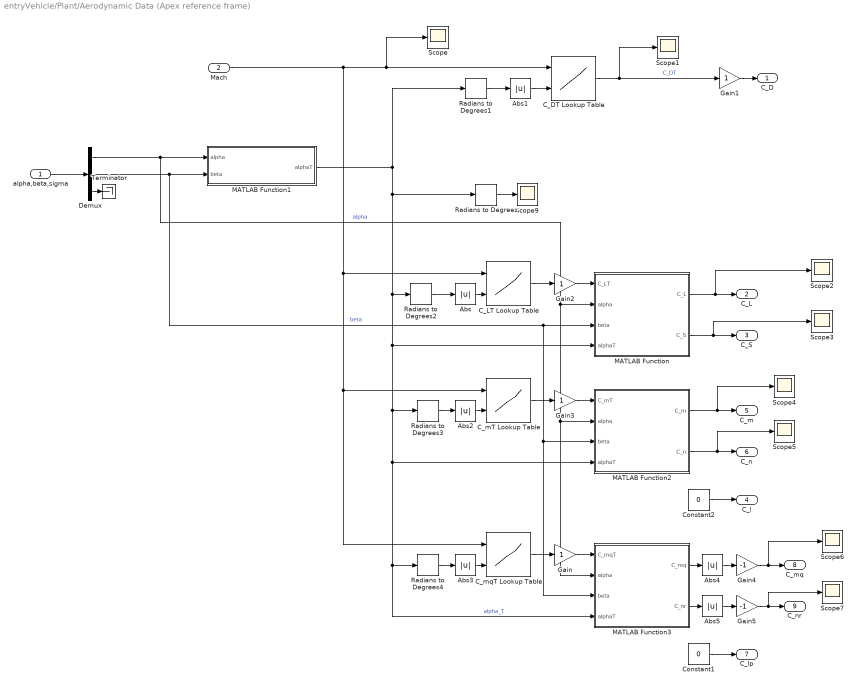
== system entryVehicle/Plant/Aerodynamic Data (Apex reference frame) ==
  alpha,beta,sigma : Inport
  Mach : Inport  Port=2
  Abs{,1..5} (6 alike) : Abs  SaturateOnIntegerOverflow=off
  C_DT Lookup Table : Lookup_n-D  BreakpointsForDimension1=Mach_numbers_CD  BreakpointsForDimension2=alpha_T_CD  Table=CD_T  ExtrapMethod=Clip  InternalRulePriority=Speed  RndMeth=Simplest
      settings: InputPortMap=u0,u1
  C_LT Lookup Table : Lookup_n-D  BreakpointsForDimension1=Mach_numbers_CL  BreakpointsForDimension2=alpha_T_CL  Table=CL_T  ExtrapMethod=Clip  InternalRulePriority=Speed  RndMeth=Simplest
      settings: InputPortMap=u0,u1
  C_mT Lookup Table : Lookup_n-D  BreakpointsForDimension1=Mach_numbers_Cm  BreakpointsForDimension2=alpha_T_Cm  Table=Cm_T  ExtrapMethod=Clip  InternalRulePriority=Speed  RndMeth=Simplest
      settings: InputPortMap=u0,u1
  C_mqT Lookup Table : Lookup_n-D  BreakpointsForDimension1=Mach_numbers_Cm_q  BreakpointsForDimension2=alpha_T_Cm_q  Table=Cm_qT  ExtrapMethod=Clip  InternalRulePriority=Speed  RndMeth=Simplest
      settings: InputPortMap=u0,u1
  Constant1 : Constant  Value=0  SampleTime=stepTime
  Constant2 : Constant  Value=0  SampleTime=stepTime
  Demux : Demux  Outputs=3
  Gain{,1..3} (4 alike) : Gain
  Gain4 : Gain  Gain=-1
  Gain5 : Gain  Gain=-1
  MATLAB Function : MATLAB Function  TreatAsAtomicUnit=on
  MATLAB Function1 : MATLAB Function  TreatAsAtomicUnit=on
  MATLAB Function2 : MATLAB Function  TreatAsAtomicUnit=on
  MATLAB Function3 : MATLAB Function  TreatAsAtomicUnit=on
  Radians to Degrees{,1..4} (5 alike) : simulink_extras/Transformations/Radians to Degrees
  Scope{,1..7,9} (9 alike) : Scope
  Terminator : Terminator
  C_D : Outport
  C_L : Outport  Port=2
  C_S : Outport  Port=3
  C_l : Outport  Port=4
  C_m : Outport  Port=5
  C_n : Outport  Port=6
  C_lp : Outport  Port=7
  C_mq : Outport  Port=8
  C_nr : Outport  Port=9
  wires:
  alpha,beta,sigma/1 -> Demux/1
  Demux/1 -> MATLAB Function1/1(alpha), MATLAB Function3/2(alpha), MATLAB Function2/2(alpha), MATLAB Function/2(alpha)  "alpha"
  Demux/2 -> MATLAB Function1/2(beta), MATLAB Function/3(beta), MATLAB Function3/3(beta), MATLAB Function2/3(beta)  "beta"
  Demux/3 -> Terminator/1
  Constant2/1 -> C_l/1
  MATLAB Function1/1(alphaT) -> Radians to Degrees1/1, Radians to Degrees/1, Radians to Degrees2/1, MATLAB Function/4(alphaT), Radians to Degrees3/1, MATLAB Function2/4(alphaT), Radians to Degrees4/1, MATLAB Function3/4(alphaT)  "alpha_T"
  C_DT Lookup Table/1 -> Gain1/1, Scope1/1  "C_DT"
  MATLAB Function/1(C_L) -> Scope2/1, C_L/1
  MATLAB Function/2(C_S) -> Scope3/1, C_S/1
  C_mT Lookup Table/1 -> Gain3/1
  MATLAB Function2/1(C_m) -> C_m/1, Scope4/1
  MATLAB Function2/2(C_n) -> Scope5/1, C_n/1
  MATLAB Function3/2(C_nr) -> Abs5/1
  MATLAB Function3/1(C_mq) -> Abs4/1
  Constant1/1 -> C_lp/1
  Abs/1 -> C_LT Lookup Table/2
  Abs1/1 -> C_DT Lookup Table/2
  Abs3/1 -> C_mqT Lookup Table/2
  Abs2/1 -> C_mT Lookup Table/2
  Radians to Degrees/1 -> Scope9/1
  Radians to Degrees1/1 -> Abs1/1
  Radians to Degrees2/1 -> Abs/1
  Radians to Degrees3/1 -> Abs2/1
  Radians to Degrees4/1 -> Abs3/1
  C_LT Lookup Table/1 -> Gain2/1
  Mach/1 -> Scope/1, C_DT Lookup Table/1, C_mqT Lookup Table/1, C_mT Lookup Table/1, C_LT Lookup Table/1
  C_mqT Lookup Table/1 -> Gain/1
  Gain/1 -> MATLAB Function3/1(C_mqT)
  Gain1/1 -> C_D/1
  Gain2/1 -> MATLAB Function/1(C_LT)
  Gain3/1 -> MATLAB Function2/1(C_mT)
  Abs4/1 -> Gain4/1
  Gain4/1 -> C_mq/1, Scope6/1
  Abs5/1 -> Gain5/1
  Gain5/1 -> C_nr/1, Scope7/1

== system entryVehicle/Plant/Altitude ==
  R,tau,lambda : Inport
  Constant : Constant  Value=Mars_radius  SampleTime=stepTime
  Demux : Demux  Outputs=3
  Sum : Sum  Inputs=|+-
  Terminator : Terminator
  Terminator1 : Terminator
  h : Outport
  wires:
  Constant/1 -> Sum/2
  Sum/1 -> h/1
  Demux/1 -> Sum/1  "R"
  R,tau,lambda/1 -> Demux/1
  Demux/2 -> Terminator/1
  Demux/3 -> Terminator1/1

== system entryVehicle/Plant/Atmosphere ==
  h : Inport
  Atmospheric Density : Subsystem
  Constant : Constant  Value=288  SampleTime=stepTime
  Scope : Scope
  To Workspace : ToWorkspace  VariableName=rho  SaveFormat=Structure With Time  SampleTime=-1
  rho : Outport
  T : Outport  Port=2
  wires:
  h/1 -> Atmospheric Density/1(h)
  Atmospheric Density/1(rho) -> To Workspace/1, Scope/1, rho/1
  Constant/1 -> T/1

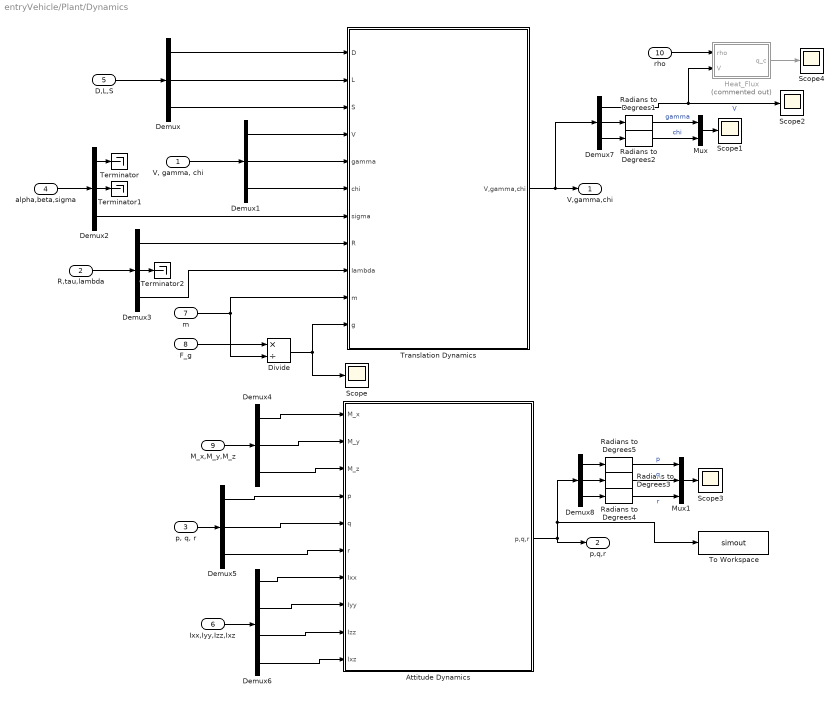
== system entryVehicle/Plant/Dynamics ==
  "V, gamma, chi" : Inport
  R,tau,lambda : Inport  Port=2
  "p, q, r" : Inport  Port=3
  alpha,beta,sigma : Inport  Port=4
  D,L,S : Inport  Port=5
  Ixx,Iyy,Izz,Ixz : Inport  Port=6
  m : Inport  Port=7
  F_g : Inport  Port=8
  M_x,M_y,M_z : Inport  Port=9
  rho : Inport  Port=10
  Attitude Dynamics : Subsystem
  Demux{,1..5,7..8} (8 alike) : Demux  Outputs=3
  Demux6 : Demux
  Divide : Product  Inputs=*/
  Heat_Flux : Subsystem  Commented=on
  Mux : Mux  Inputs=2
  Mux1 : Mux  Inputs=3
  Radians to Degrees{1..5} (5 alike) : simulink_extras/Transformations/Radians to Degrees
  Scope{,1..4} (5 alike) : Scope
  Terminator : Terminator
  Terminator1 : Terminator
  Terminator2 : Terminator
  To Workspace : ToWorkspace  VariableName=simout  SaveFormat=Structure With Time  SampleTime=-1
  Translation Dynamics : Subsystem
  V,gamma,chi : Outport
  p,q,r : Outport  Port=2
  wires:
  Translation Dynamics/1(V,gamma,chi) -> Demux7/1, V,gamma,chi/1
  Attitude Dynamics/1(p,q,r) -> p,q,r/1, Demux8/1, To Workspace/1
  Demux/2 -> Translation Dynamics/2(L)
  Demux/1 -> Translation Dynamics/1(D)
  Demux/3 -> Translation Dynamics/3(S)
  D,L,S/1 -> Demux/1
  "V, gamma, chi"/1 -> Demux1/1
  Demux1/1 -> Translation Dynamics/4(V)
  Demux1/2 -> Translation Dynamics/5(gamma)
  Demux1/3 -> Translation Dynamics/6(chi)
  alpha,beta,sigma/1 -> Demux2/1
  Demux2/3 -> Translation Dynamics/7(sigma)
  Demux2/1 -> Terminator/1
  Demux2/2 -> Terminator1/1
  R,tau,lambda/1 -> Demux3/1
  Demux3/1 -> Translation Dynamics/8(R)
  Demux3/3 -> Translation Dynamics/9(lambda)
  Demux3/2 -> Terminator2/1
  Demux4/2 -> Attitude Dynamics/2(M_y)
  Demux4/1 -> Attitude Dynamics/1(M_x)
  Demux4/3 -> Attitude Dynamics/3(M_z)
  M_x,M_y,M_z/1 -> Demux4/1
  "p, q, r"/1 -> Demux5/1
  Demux5/1 -> Attitude Dynamics/4(p)
  Demux5/2 -> Attitude Dynamics/5(q)
  Demux5/3 -> Attitude Dynamics/6(r)
  Demux6/1 -> Attitude Dynamics/7(Ixx)
  Demux6/2 -> Attitude Dynamics/8(Iyy)
  Demux6/3 -> Attitude Dynamics/9(Izz)
  Ixx,Iyy,Izz,Ixz/1 -> Demux6/1
  Demux6/4 -> Attitude Dynamics/10(Ixz)
  m/1 -> Divide/2, Translation Dynamics/10(m)
  Divide/1 -> Scope/1, Translation Dynamics/11(g)
  F_g/1 -> Divide/1
  Radians to Degrees4/1 -> Mux1/3  "r"
  Demux8/2 -> Radians to Degrees3/1
  Demux8/1 -> Radians to Degrees5/1
  Mux1/1 -> Scope3/1
  Radians to Degrees3/1 -> Mux1/2  "q"
  Radians to Degrees5/1 -> Mux1/1  "p"
  Demux8/3 -> Radians to Degrees4/1
  Radians to Degrees2/1 -> Mux/2  "chi"
  Demux7/3 -> Radians to Degrees2/1
  Demux7/1 -> Heat_Flux/2(V), Scope2/1  "V"
  Demux7/2 -> Radians to Degrees1/1
  Radians to Degrees1/1 -> Mux/1  "gamma"
  Mux/1 -> Scope1/1
  rho/1 -> Heat_Flux/1(rho)
  Heat_Flux/1(q_c) -> Scope4/1

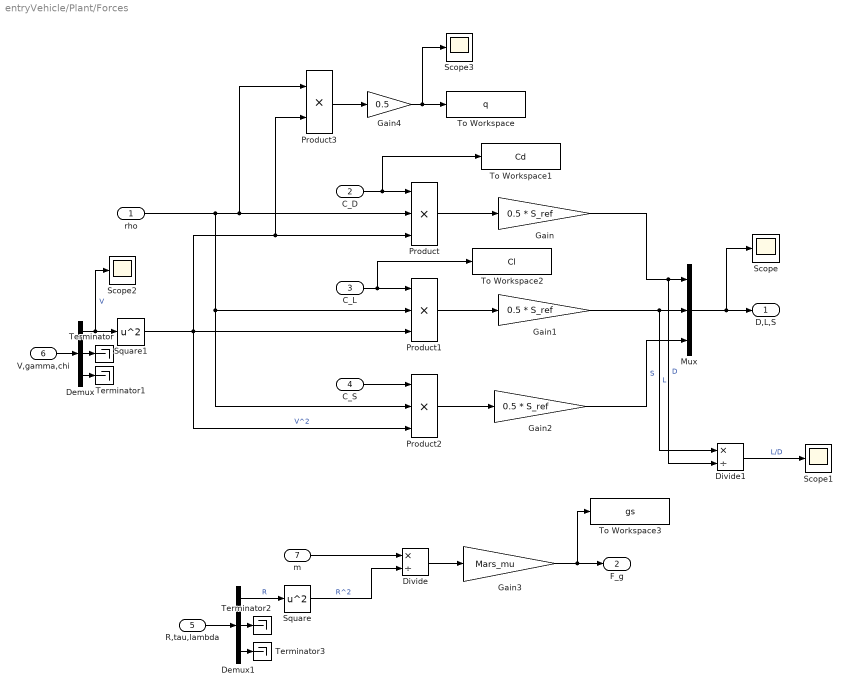
== system entryVehicle/Plant/Forces ==
  rho : Inport
  C_D : Inport  Port=2
  C_L : Inport  Port=3
  C_S : Inport  Port=4
  R,tau,lambda : Inport  Port=5
  V,gamma,chi : Inport  Port=6
  m : Inport  Port=7
  Demux : Demux  Outputs=3
  Demux1 : Demux  Outputs=3
  Divide : Product  Inputs=*/
  Divide1 : Product  Inputs=*/
  Gain : Gain  Gain=0.5 * S_ref
  Gain1 : Gain  Gain=0.5 * S_ref
  Gain2 : Gain  Gain=0.5 * S_ref
  Gain3 : Gain  Gain=Mars_mu
  Gain4 : Gain  Gain=0.5
  Mux : Mux  Inputs=3
  Product : Product  Inputs=3
  Product1 : Product  Inputs=3
  Product2 : Product  Inputs=3
  Product3 : Product
  Scope{,1..3} (4 alike) : Scope
  Square : Math  Operator=square  OutputSignalType=real
  Square1 : Math  Operator=square
  Terminator{,1..3} (4 alike) : Terminator
  To Workspace : ToWorkspace  VariableName=q  SaveFormat=Structure With Time  SampleTime=-1
  To Workspace1 : ToWorkspace  VariableName=Cd  SaveFormat=Structure With Time  SampleTime=-1
  To Workspace2 : ToWorkspace  VariableName=Cl  SaveFormat=Structure With Time  SampleTime=-1
  To Workspace3 : ToWorkspace  VariableName=gs  SaveFormat=Structure With Time  SampleTime=-1
  D,L,S : Outport
  F_g : Outport  Port=2
  wires:
  C_D/1 -> To Workspace1/1, Product/1
  rho/1 -> Product2/2, Product1/2, Product/2, Product3/1
  V,gamma,chi/1 -> Demux/1
  Demux/2 -> Terminator/1
  Demux/3 -> Terminator1/1
  Product/1 -> Gain/1
  C_L/1 -> To Workspace2/1, Product1/1
  C_S/1 -> Product2/1
  Product1/1 -> Gain1/1
  Product2/1 -> Gain2/1
  Gain1/1 -> Divide1/1, Mux/2  "L"
  Gain/1 -> Mux/1, Divide1/2  "D"
  Gain2/1 -> Mux/3  "S"
  Mux/1 -> D,L,S/1, Scope/1
  Demux1/2 -> Terminator2/1
  Demux1/3 -> Terminator3/1
  R,tau,lambda/1 -> Demux1/1
  m/1 -> Divide/1
  Divide/1 -> Gain3/1
  Gain3/1 -> To Workspace3/1, F_g/1
  Demux1/1 -> Square/1  "R"
  Square/1 -> Divide/2  "R^2"
  Demux/1 -> Scope2/1, Square1/1  "V"
  Square1/1 -> Product2/3, Product/3, Product3/2, Product1/3  "V^2"
  Divide1/1 -> Scope1/1  "L/D"
  Product3/1 -> Gain4/1
  Gain4/1 -> To Workspace/1, Scope3/1

== system entryVehicle/Plant/Fuel ==
  Mtx : Inport
  Impulse : Scope
  Integrator : Integrator
  To Workspace4 : ToWorkspace  VariableName=impulse  SaveFormat=Timeseries  SampleTime=-1
  wires:
  Integrator/1 -> To Workspace4/1, Impulse/1
  Mtx/1 -> Integrator/1

== system entryVehicle/Plant/Ground Colision Check ==
  h : Inport
  Constant : Constant  Value=0  SampleTime=stepTime
  Constant1 : Constant  SampleTime=stepTime
  Stop Simulation : Stop
  Switch : Switch  SaturateOnIntegerOverflow=off  InputSameDT=off
  wires:
  Switch/1 -> Stop Simulation/1
  Constant/1 -> Switch/1
  Constant1/1 -> Switch/3
  h/1 -> Switch/2

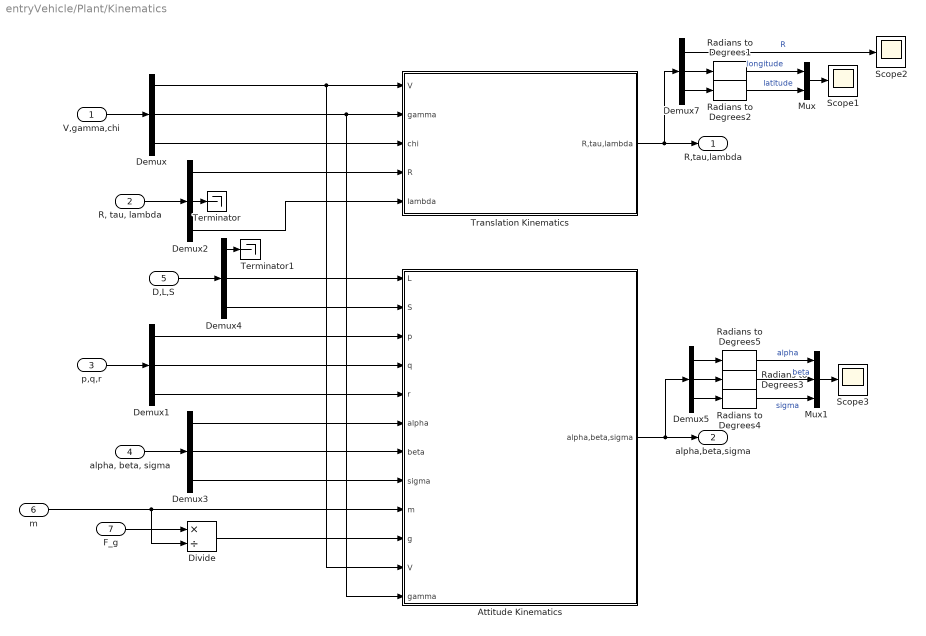
== system entryVehicle/Plant/Kinematics ==
  V,gamma,chi : Inport
  "R, tau, lambda" : Inport  Port=2
  p,q,r : Inport  Port=3
  "alpha, beta, sigma" : Inport  Port=4
  D,L,S : Inport  Port=5
  m : Inport  Port=6
  F_g : Inport  Port=7
  Attitude Kinematics : Subsystem
  Demux{,1..5,7} (7 alike) : Demux  Outputs=3
  Divide : Product  Inputs=*/
  Mux : Mux  Inputs=2
  Mux1 : Mux  Inputs=3
  Radians to Degrees{1..5} (5 alike) : simulink_extras/Transformations/Radians to Degrees
  Scope1 : Scope
  Scope2 : Scope
  Scope3 : Scope
  Terminator : Terminator
  Terminator1 : Terminator
  Translation Kinematics : Subsystem
  R,tau,lambda : Outport
  alpha,beta,sigma : Outport  Port=2
  wires:
  Translation Kinematics/1(R,tau,lambda) -> Demux7/1, R,tau,lambda/1
  Attitude Kinematics/1(alpha,beta,sigma) -> Demux5/1, alpha,beta,sigma/1
  V,gamma,chi/1 -> Demux/1
  Demux/1 -> Translation Kinematics/1(V), Attitude Kinematics/11(V)
  Demux/2 -> Attitude Kinematics/12(gamma), Translation Kinematics/2(gamma)
  Demux/3 -> Translation Kinematics/3(chi)
  p,q,r/1 -> Demux1/1
  Demux1/1 -> Attitude Kinematics/3(p)
  Demux1/2 -> Attitude Kinematics/4(q)
  Demux1/3 -> Attitude Kinematics/5(r)
  "R, tau, lambda"/1 -> Demux2/1
  Demux2/1 -> Translation Kinematics/4(R)
  Demux2/3 -> Translation Kinematics/5(lambda)
  Demux3/2 -> Attitude Kinematics/7(beta)
  Demux3/1 -> Attitude Kinematics/6(alpha)
  Demux3/3 -> Attitude Kinematics/8(sigma)
  "alpha, beta, sigma"/1 -> Demux3/1
  m/1 -> Divide/2, Attitude Kinematics/9(m)
  Divide/1 -> Attitude Kinematics/10(g)
  F_g/1 -> Divide/1
  Demux2/2 -> Terminator/1
  D,L,S/1 -> Demux4/1
  Demux4/2 -> Attitude Kinematics/1(L)
  Demux4/3 -> Attitude Kinematics/2(S)
  Demux4/1 -> Terminator1/1
  Mux/1 -> Scope1/1
  Demux7/1 -> Scope2/1  "R"
  Demux7/2 -> Radians to Degrees1/1
  Demux7/3 -> Radians to Degrees2/1
  Radians to Degrees2/1 -> Mux/2  "latitude"
  Radians to Degrees1/1 -> Mux/1  "longitude"
  Radians to Degrees4/1 -> Mux1/3  "sigma"
  Demux5/3 -> Radians to Degrees4/1
  Demux5/2 -> Radians to Degrees3/1
  Radians to Degrees3/1 -> Mux1/2  "beta"
  Mux1/1 -> Scope3/1
  Demux5/1 -> Radians to Degrees5/1
  Radians to Degrees5/1 -> Mux1/1  "alpha"

== system entryVehicle/Plant/Mach Number ==
  T : Inport
  V,gamma,chi : Inport  Port=2
  Constant : Constant  Value=5
  Demux : Demux  Outputs=3
  Divide : Product  Inputs=*/
  Gain : Gain  Gain=specific_heat * R_s
  Manual Switch : ManualSwitch  CurrentSetting=0
  Scope : Scope
  Scope1 : Scope
  Square Root : Sqrt  OutputSignalType=real
  Terminator : Terminator
  Terminator1 : Terminator
  Mach : Outport
  wires:
  V,gamma,chi/1 -> Demux/1
  Demux/3 -> Terminator/1
  Demux/2 -> Terminator1/1
  Demux/1 -> Divide/1  "V"
  Square Root/1 -> Scope/1, Divide/2  "a"
  T/1 -> Gain/1
  Gain/1 -> Square Root/1
  Divide/1 -> Manual Switch/2
  Manual Switch/1 -> Scope1/1, Mach/1
  Constant/1 -> Manual Switch/1

== system entryVehicle/Plant/Mass Properties ==
  Constant : Constant  Value=m_0  SampleTime=stepTime
  Constant1 : Constant  Value=I_xx  SampleTime=stepTime
  Constant2 : Constant  Value=I_yy  SampleTime=stepTime
  Constant3 : Constant  Value=I_zz  SampleTime=stepTime
  Constant4 : Constant  Value=I_xz  SampleTime=stepTime
  Mux : Mux
  m : Outport
  I_xx,I_yy,I_zz,I_xz : Outport  Port=2
  wires:
  Constant/1 -> m/1
  Constant2/1 -> Mux/2
  Constant3/1 -> Mux/3
  Constant1/1 -> Mux/1
  Constant4/1 -> Mux/4
  Mux/1 -> I_xx,I_yy,I_zz,I_xz/1

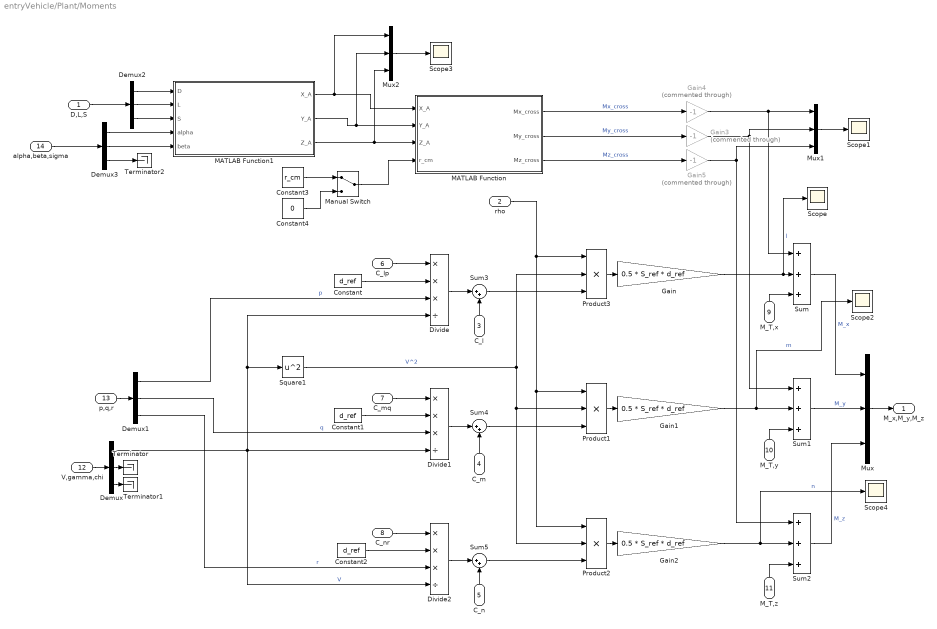
== system entryVehicle/Plant/Moments ==
  D,L,S : Inport
  rho : Inport  Port=2
  C_l : Inport  Port=3
  C_m : Inport  Port=4
  C_n : Inport  Port=5
  C_lp : Inport  Port=6
  C_mq : Inport  Port=7
  C_nr : Inport  Port=8
  M_T,x : Inport  Port=9
  M_T,y : Inport  Port=10
  M_T,z : Inport  Port=11
  V,gamma,chi : Inport  Port=12
  p,q,r : Inport  Port=13
  alpha,beta,sigma : Inport  Port=14
  Constant : Constant  Value=d_ref  SampleTime=stepTime
  Constant1 : Constant  Value=d_ref  SampleTime=stepTime
  Constant2 : Constant  Value=d_ref  SampleTime=stepTime
  Constant3 : Constant  Value=r_cm
  Constant4 : Constant  Value=0
  Demux{,1..3} (4 alike) : Demux  Outputs=3
  Divide : Product  Inputs=***/
  Divide1 : Product  Inputs=***/
  Divide2 : Product  Inputs=***/
  Gain : Gain  Gain=0.5 * S_ref * d_ref
  Gain1 : Gain  Gain=0.5 * S_ref * d_ref
  Gain2 : Gain  Gain=0.5 * S_ref * d_ref
  Gain3 : Gain  Commented=through  Gain=-1
  Gain4 : Gain  Commented=through  Gain=-1
  Gain5 : Gain  Commented=through  Gain=-1
  MATLAB Function : MATLAB Function  TreatAsAtomicUnit=on
  MATLAB Function1 : MATLAB Function  TreatAsAtomicUnit=on
  Manual Switch : ManualSwitch
  Mux : Mux  Inputs=3
  Mux1 : Mux  Inputs=3
  Mux2 : Mux  Inputs=3
  Product1 : Product  Inputs=3
  Product2 : Product  Inputs=3
  Product3 : Product  Inputs=3
  Scope{,1..4} (5 alike) : Scope
  Square1 : Math  Operator=square
  Sum : Sum  Inputs=+|+|+
  Sum1 : Sum  Inputs=+|+|+
  Sum2 : Sum  Inputs=+|+|+
  Sum3 : Sum  Inputs=|++
  Sum4 : Sum  Inputs=|++
  Sum5 : Sum  Inputs=|++
  Terminator : Terminator
  Terminator1 : Terminator
  Terminator2 : Terminator
  M_x,M_y,M_z : Outport
  wires:
  Gain2/1 -> Scope4/1, Sum2/2  "n"
  V,gamma,chi/1 -> Demux/1
  Gain1/1 -> Scope2/1, Sum1/2  "m"
  Gain/1 -> Scope/1, Sum/2  "l"
  Demux/3 -> Terminator1/1
  Demux/1 -> Divide2/4, Divide1/4, Divide/4, Square1/1  "V"
  Product1/1 -> Gain1/1
  Demux/2 -> Terminator/1
  Product2/1 -> Gain2/1
  M_T,x/1 -> Sum/3
  M_T,y/1 -> Sum1/3
  M_T,z/1 -> Sum2/3
  Sum1/1 -> Mux/2  "M_y"
  Sum/1 -> Mux/1  "M_x"
  Sum2/1 -> Mux/3  "M_z"
  Mux/1 -> M_x,M_y,M_z/1
  p,q,r/1 -> Demux1/1
  Product3/1 -> Gain/1
  C_l/1 -> Sum3/2
  C_lp/1 -> Divide/1
  Demux1/1 -> Divide/3  "p"
  Sum3/1 -> Product3/3
  Divide/1 -> Sum3/1
  Constant/1 -> Divide/2
  rho/1 -> Product3/1, Product2/1, Product1/1
  Divide1/1 -> Sum4/1
  Sum4/1 -> Product1/3
  C_m/1 -> Sum4/2
  Divide2/1 -> Sum5/1
  Sum5/1 -> Product2/3
  C_n/1 -> Sum5/2
  C_mq/1 -> Divide1/1
  C_nr/1 -> Divide2/1
  Constant1/1 -> Divide1/2
  Constant2/1 -> Divide2/2
  Square1/1 -> Product2/2, Product1/2, Product3/2  "V^2"
  Demux1/2 -> Divide1/3  "q"
  Demux1/3 -> Divide2/3  "r"
  D,L,S/1 -> Demux2/1
  Manual Switch/1 -> MATLAB Function/4(r_cm)
  MATLAB Function/1(Mx_cross) -> Gain4/1  "Mx_cross"
  MATLAB Function/2(My_cross) -> Gain3/1  "My_cross"
  MATLAB Function/3(Mz_cross) -> Gain5/1  "Mz_cross"
  Constant3/1 -> Manual Switch/1
  Constant4/1 -> Manual Switch/2
  Demux2/1 -> MATLAB Function1/1(D)
  Demux2/2 -> MATLAB Function1/2(L)
  Demux2/3 -> MATLAB Function1/3(S)
  Demux3/1 -> MATLAB Function1/4(alpha)
  Demux3/2 -> MATLAB Function1/5(beta)
  alpha,beta,sigma/1 -> Demux3/1
  Demux3/3 -> Terminator2/1
  MATLAB Function1/1(X_A) -> MATLAB Function/1(X_A), Mux2/1
  MATLAB Function1/2(Y_A) -> MATLAB Function/2(Y_A), Mux2/2
  MATLAB Function1/3(Z_A) -> Mux2/3, MATLAB Function/3(Z_A)
  Mux1/1 -> Scope1/1
  Mux2/1 -> Scope3/1
  Gain3/1 -> Mux1/2, Sum1/1
  Gain4/1 -> Mux1/1, Sum/1
  Gain5/1 -> Mux1/3, Sum2/1

== system entryVehicle/Plant/state ==
  R,tau,delta : Inport
  alpha,beta,sigma : Inport  Port=2
  V,gamma,chi : Inport  Port=3
  p,q,r : Inport  Port=4
  Mux : Mux
  state : Outport
  wires:
  Mux/1 -> state/1
  R,tau,delta/1 -> Mux/1
  alpha,beta,sigma/1 -> Mux/2
  V,gamma,chi/1 -> Mux/3
  p,q,r/1 -> Mux/4

== system entryVehicle/State Space/Lateral_Controller ==
  lateral_state : Inport
  lateral_ref : Inport  Port=2
  Gain : Gain  Gain=-K_lat  Multiplication=Matrix(K*u)
  Sum : Sum  Inputs=|+-
  Mx,Mtz : Outport
  wires:
  lateral_ref/1 -> Sum/2
  Sum/1 -> Gain/1
  lateral_state/1 -> Sum/1
  Gain/1 -> Mx,Mtz/1

== system entryVehicle/State Space/Longitudinal_Controller ==
  longitudinal : Inport
  longitudinal_ref : Inport  Port=2
  Gain : Gain  Gain=-K_long  Multiplication=Matrix(K*u)
  Sum : Sum  Inputs=|+-
  My : Outport
  wires:
  longitudinal_ref/1 -> Sum/2
  Sum/1 -> Gain/1
  longitudinal/1 -> Sum/1
  Gain/1 -> My/1
